simulink model "PUIOaugModel"  (R2017a)
settings: Solver=VariableStepAuto  StartTime=0.0  StopTime=tEnd  RelTol=1e-3  EnableMultiTasking=on
values from neighbouring files (symbols this model uses):
  Aaug = [A, zeros(n,p);Maug*C, -Maug]    [ExampleActuatorSensor.m]    (also in Untitled.m)
  Baug = [B;zeros(p,m)]    [ExampleActuatorSensor.m]    (also in Untitled.m)
  Caug = [C,eye(p,p)]    [ExampleActuatorSensor.m]    (also in Untitled.m)
  Eaug = [Ea,zeros(n,qs);zeros(p,qa),Maug*Es]    [ExampleActuatorSensor.m]    (also in Untitled.m)
  F = A1 - G1*C    [ExampleActuator.m]    (also in ExampleActuatorSensor.m = A1 - G1*Caug; ExamplePIUIO.m = A1-G1*C; SinousidPIUIO.m = A1-G1*C; Untitled.m = A1 - G1*Caug)
  faug = faugTS.Values.Data    [ExampleActuatorSensor.m]    (also in Untitled.m)
  G = G1 + A1*N - G1*C*N    [ExampleActuator.m]    (also in ExampleActuatorSensor.m = G1 + A1*N - G1*Caug*N; ExamplePIUIO.m = G1+G2; SinousidPIUIO.m = G1+G2; Untitled.m = G1 + A1*N - G1*Caug*N)
  H = T*B    [ExampleActuator.m]    (also in ExampleActuatorSensor.m = T*Baug; ExamplePIUIO.m; SinousidPIUIO.m; Untitled.m = T*Baug)
  M = eye(size(A))    [ExampleActuator.m]    (also in ExampleActuatorSensor.m = eye(size(Aaug)); Untitled.m = eye(size(Aaug)))
  N = Ed* pinv(C*Ed)    [ExampleActuator.m]    (also in ExampleActuatorSensor.m = Eaug* pinv(Caug*Eaug); ExamplePIUIO.m; SinousidPIUIO.m; Untitled.m = Eaug* pinv(Caug*Eaug))
  Ndhat = pinv(C*Ed)    [ExampleActuator.m]    (also in ExampleActuatorSensor.m = pinv(Caug*Eaug); Untitled.m = pinv(Caug*Eaug))
  x0aug = [x0;v0]    [ExampleActuatorSensor.m]    (also in Untitled.m)
  z0 = [0.1;0.2;0.3]    [ExampleActuator.m]    (also in ExampleActuatorSensor.m = [0.1;.2;.3;0.4;0.5]; ExamplePIUIO.m = xhat0; SinousidPIUIO.m = xhat0; Untitled.m = [0.1;0.2;0.3;0.4;0.5])
settings Model: Creator=amirreza513  LastModifiedBy=amirreza513
settings OptimizationCC: LifeSpan=inf
settings DebuggingCC: SFUnexpectedBacktrackingDiag=warning  SFNoUnconditionalDefaultTransitionDiag=warning  SFExecutionAtInitializationDiag=none
settings GRTTargetCC: TargetLangStandard=C89/C90 (ANSI)  GeneratePreprocessorConditionals=Disable all
settings ConfigComp: CovMetricSettings=dw  CovHtmlReporting=on  CovSaveCumulativeToWorkspaceVar=on  CovSaveSingleToWorkspaceVar=on  CovExternalEMLEnable=off

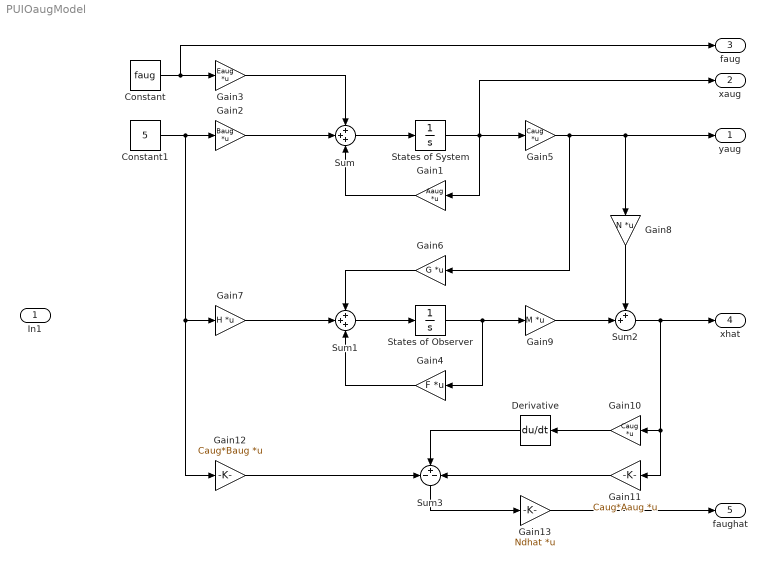
== system PUIOaugModel ==
  In1 : Inport
  Constant : Constant  Value=faug
  Constant1 : Constant  Value=5
  Derivative : Derivative  CoefficientInTFapproximation=0
  Gain1 : Gain  Gain=Aaug  Multiplication=Matrix(K*u) (u vector)
  Gain10 : Gain  Gain=Caug  Multiplication=Matrix(K*u) (u vector)
  Gain11 : Gain  Gain=Caug*Aaug  Multiplication=Matrix(K*u) (u vector)
  Gain12 : Gain  Gain=Caug*Baug  Multiplication=Matrix(K*u) (u vector)
  Gain13 : Gain  Gain=Ndhat  Multiplication=Matrix(K*u) (u vector)
  Gain2 : Gain  Gain=Baug  Multiplication=Matrix(K*u) (u vector)
  Gain3 : Gain  Gain=Eaug  Multiplication=Matrix(K*u) (u vector)
  Gain4 : Gain  Gain=F  Multiplication=Matrix(K*u) (u vector)
  Gain5 : Gain  Gain=Caug  Multiplication=Matrix(K*u) (u vector)
  Gain6 : Gain  Gain=G  Multiplication=Matrix(K*u) (u vector)
  Gain7 : Gain  Gain=H  Multiplication=Matrix(K*u) (u vector)
  Gain8 : Gain  Gain=N  Multiplication=Matrix(K*u) (u vector)
  Gain9 : Gain  Gain=M  Multiplication=Matrix(K*u) (u vector)
  States of Observer : Integrator  InitialCondition=z0
  States of System : Integrator  InitialCondition=x0aug
  Sum : Sum  Inputs=+++
  Sum1 : Sum  Inputs=+++
  Sum2 : Sum  Inputs=++|
  Sum3 : Sum  Inputs=-+-
  yaug : Outport
  xaug : Outport  Port=2
  faug : Outport  Port=3
  xhat : Outport  Port=4
  faughat : Outport  Port=5
  wires:
  States of System/1 -> xaug/1, Gain5/1, Gain1/1
  Constant1/1 -> Gain12/1, Gain7/1, Gain2/1
  Gain2/1 -> Sum/2
  Constant/1 -> faug/1, Gain3/1
  Sum/1 -> States of System/1
  Gain5/1 -> Gain6/1, Gain8/1, yaug/1
  Gain3/1 -> Sum/1
  Gain1/1 -> Sum/3
  Sum1/1 -> States of Observer/1
  States of Observer/1 -> Gain9/1, Gain4/1
  Gain6/1 -> Sum1/1
  Gain7/1 -> Sum1/2
  Gain4/1 -> Sum1/3
  Gain8/1 -> Sum2/1
  Gain9/1 -> Sum2/2
  Gain10/1 -> Derivative/1
  Sum2/1 -> Gain11/1, Gain10/1, xhat/1
  Gain12/1 -> Sum3/1
  Derivative/1 -> Sum3/2
  Gain11/1 -> Sum3/3
  Sum3/1 -> Gain13/1
  Gain13/1 -> faughat/1
